simulink model "grua_portuaria"  (R2021a)
settings: Solver=VariableStepAuto  StartTime=0.0  StopTime=2  RelTol=1e-3
values from neighbouring files (symbols this model uses):
  b_cx = 1*10^6    (= 1000000)    [parametros.m]
  b_cy = 1*10^7    (= 10000000)    [parametros.m]
  b_eq = (b_td+b_tm*(r_t^2))/r_td    (= 10803.6)    [parametros.m]
  b_eqh = 2*(b_hd+b_hm*(r_h^2))/r_hd    (= 23253.3333333)    [parametros.m]
  b_ha = b_eqh/r_h - n_h*w_posh*(J_eqh + 0.5*m_l_*r_hd)/r_h    [parametros.m]
  b_hb = 1*10^8    (= 100000000)    [parametros.m]
  b_hEb = 2.2*10^9    (= 2200000000)    [parametros.m]
  b_t = 90    [parametros.m]
  b_ta = n_t*w_post*(r_td*J_eqt/r_t) - r_td*b_eqt/r_t    [parametros.m]
  b_tb = 5*10^6    (= 5000000)    [parametros.m]
  b_tw = 3*10^3    (= 3000)    [parametros.m]
  b_wu = 150    [parametros.m]
  g = 9.80665    [parametros.m]
  H_c = 2.5    [parametros.m]
  J_eq = (J_td+J_tm_tb*(r_t^2))/r_td    (= 15000)    [parametros.m]
  J_eqh = 2*(J_hd_hEb+J_hm_hb*(r_h^2))/r_hd    (= 48853.3333333)    [parametros.m]
  K_cy = 1.8*10^9    (= 1800000000)    [parametros.m]
  K_hsa = -n_h*(w_posh^2)*(J_eqh + 0.5*m_l_*r_hd)/r_t    [parametros.m]
  K_hsia = -(w_posh^3)*(J_eqh + 0.5*m_l_*r_hd)/r_t    [parametros.m]
  K_tsa = n_t*(w_post^2)*J_eqt*r_td/r_t    [parametros.m]
  K_tsia = (w_post^3)*J_eqt*r_td/r_t    [parametros.m]
  K_tw = 4.8*10^5    (= 480000)    [parametros.m]
  k_wu = 2.36*10^8    (= 236000000)    [parametros.m]
  M_s = 15000    [parametros.m]
  M_t = 30000    [parametros.m]
  r_h = 22    [parametros.m]
  r_hd = 0.75    [parametros.m]
  r_t = 30    [parametros.m]
  r_td = 0.5    [parametros.m]
  T_hb_MAX = 5*10^5    (= 500000)    [parametros.m]
  T_hEb_MAX = 1.1*10^6    (= 1100000)    [parametros.m]
  T_s2 = 5e-3    (= 0.005)    [parametros.m]
  T_tb_MAX = 5*10^4    (= 50000)    [parametros.m]
  tau_hm = 1e-3    (= 0.001)    [parametros.m]
  tau_tm = 1e-3    (= 0.001)    [parametros.m]
  Y_t0 = 45    [parametros.m]
undefined symbols (not defined in the file or in its folder): T_s
libraries: simulink x9, dspstat3 x1, vrlib x1
(part 1 of 3)
settings Model: Creator=aguss  LastModifiedBy=Usuario

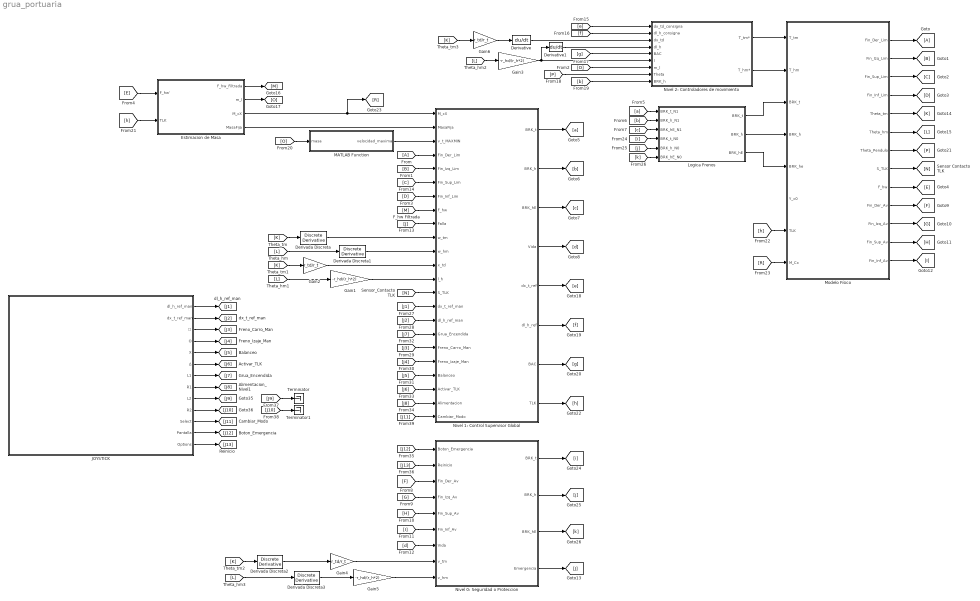
== system grua_portuaria ==
  Derivada Discreta{,1..3} (4 alike) : simulink/Discrete/Discrete Derivative  gainval=1.0  ICPrevScaledInput=0.0  OutMin=[]  OutMax=[]  OutDataType=fixdt(1, 16)  OutScaling=2^-10  DoSatur=off
  Derivative : Derivative
  Derivative1 : Derivative
  Estimacion de Masa : Subsystem
  Gain1 : Gain  Gain=-r_hd/(r_h*2)
  Gain2 : Gain  Gain=r_td/r_t
  Gain3 : Gain  Gain=-r_hd/(r_h*2)
  Gain4 : Gain  Gain=r_td/r_t
  Gain5 : Gain  Gain=-r_hd/(r_h*2)
  Gain6 : Gain  Gain=r_td/r_t
  JOYSTICK : Subsystem
  Logica Frenos : Subsystem
  MATLAB Function : MATLAB Function  TreatAsAtomicUnit=on
  Modelo Físico : Subsystem
  Nivel 0: Seguridad o Proteccion : Subsystem
  Nivel 1: Control Supervisor Global : Subsystem
  Nivel 2: Controladores de movimiento : Subsystem
  Terminator : Terminator
  Terminator1 : Terminator
  wires:
  Nivel 2: Controladores de movimiento/2(T_hm*) -> Modelo Físico/2(T_hm)
  Nivel 2: Controladores de movimiento/1(T_tm*) -> Modelo Físico/1(T_tm)
  Modelo Físico/1(Fin_Der_Lim) -> [A]
  Modelo Físico/2(Fin_Izq_Lim) -> [B]
  Modelo Físico/4(Fin_Inf_Lim) -> [D]
  Modelo Físico/3(Fin_Sup_Lim) -> [C]
  [A] -> Nivel 1: Control Supervisor Global/4(Fin_Der_Lim)
  [B] -> Nivel 1: Control Supervisor Global/5(Fin_Izq_Lim)
  [C] -> Nivel 1: Control Supervisor Global/6(Fin_Sup_Lim)
  [D] -> Nivel 1: Control Supervisor Global/7(Fin_Inf_Lim)
  Modelo Físico/9(F_hw) -> [E]
  Nivel 1: Control Supervisor Global/1(BRK_t) -> [a]
  Nivel 1: Control Supervisor Global/2(BRK_h) -> [b]
  Nivel 1: Control Supervisor Global/3(BRK_hE) -> [c]
  Nivel 1: Control Supervisor Global/4(Vida) -> [d]
  Modelo Físico/10(Fin_Der_Av) -> [F]
  Modelo Físico/11(Fin_Izq_Av) -> [G]
  Modelo Físico/12(Fin_Sup_Av) -> [H]
  Modelo Físico/13(Fin_Inf_Av) -> [I]
  [H] -> Nivel 0: Seguridad o Proteccion/5(Fin_Sup_Av)
  [F] -> Nivel 0: Seguridad o Proteccion/3(Fin_Der_Av)
  [G] -> Nivel 0: Seguridad o Proteccion/4(Fin_Izq_Av)
  [I] -> Nivel 0: Seguridad o Proteccion/6(Fin_Inf_Av)
  [d] -> Nivel 0: Seguridad o Proteccion/7(Vida)
  [E] -> Estimacion de Masa/1(F_hw')
  [M] -> Nivel 1: Control Supervisor Global/8(F_hw)
  Nivel 0: Seguridad o Proteccion/4(Emergencia) -> [J]
  [J] -> Nivel 1: Control Supervisor Global/9(Falla)
  Modelo Físico/5(Theta_tm) -> [K]
  [K] -> Derivada Discreta/1
  Derivada Discreta/1 -> Nivel 1: Control Supervisor Global/10(w_tm)
  Modelo Físico/6(Theta_hm) -> [L]
  [L] -> Derivada Discreta1/1
  Derivada Discreta1/1 -> Nivel 1: Control Supervisor Global/11(w_hm)
  [K] -> Gain2/1
  Gain2/1 -> Nivel 1: Control Supervisor Global/12(x_td)
  [L] -> Gain1/1
  Gain1/1 -> Nivel 1: Control Supervisor Global/13(l_h)
  Estimacion de Masa/4(MasaFija) -> Nivel 1: Control Supervisor Global/2(MasaFija)
  Estimacion de Masa/3(M_cX) -> [R], Nivel 1: Control Supervisor Global/1(M_cX)
  Estimacion de Masa/1(F_hw_Filtrada) -> [M]
  Modelo Físico/8(S_TLK) -> [N]
  [N] -> Nivel 1: Control Supervisor Global/14(S_TLK)
  Estimacion de Masa/2(m_l) -> [O]
  [O] -> Nivel 2: Controladores de movimiento/7(m_l)
  Nivel 1: Control Supervisor Global/5(dx_t_ref) -> [e]
  Nivel 1: Control Supervisor Global/6(dl_h_ref) -> [f]
  Nivel 1: Control Supervisor Global/7(BAC) -> [g]
  [g] -> Nivel 2: Controladores de movimiento/5(BAC)
  [L] -> Gain3/1
  Gain3/1 -> Nivel 2: Controladores de movimiento/6(l), Derivative1/1
  Modelo Físico/7(Theta_Pendulo) -> [P]
  [P] -> Nivel 2: Controladores de movimiento/8(Theta)
  [b] -> Nivel 2: Controladores de movimiento/9(BRK_h)
  MATLAB Function/1(velocidad_maxima) -> Nivel 1: Control Supervisor Global/3(v_t_MAXMIN)
  [O] -> MATLAB Function/1(masa)
  Nivel 1: Control Supervisor Global/8(TLK) -> [h]
  [h] -> Estimacion de Masa/2(TLK)
  [h] -> Modelo Físico/7(TLK)
  [R] -> Modelo Físico/8(M_Cx)
  [a] -> Logica Frenos/1(BRK_t_N1)
  [b] -> Logica Frenos/2(BRK_h_N1)
  [c] -> Logica Frenos/3(BRK_hE_N1)
  Nivel 0: Seguridad o Proteccion/3(BRK_hE) -> [k]
  Nivel 0: Seguridad o Proteccion/2(BRK_h) -> [j]
  Nivel 0: Seguridad o Proteccion/1(BRK_t) -> [i]
  [i] -> Logica Frenos/4(BRK_t_N0)
  [j] -> Logica Frenos/5(BRK_h_N0)
  [k] -> Logica Frenos/6(BRK_hE_N0)
  Logica Frenos/2(BRK_h) -> Modelo Físico/4(BRK_h)
  Logica Frenos/3(BRK_hE) -> Modelo Físico/5(BRK_he)
  Logica Frenos/1(BRK_t) -> Modelo Físico/3(BRK_t)
  [L] -> Derivada Discreta3/1
  Derivada Discreta2/1 -> Gain4/1
  [K] -> Derivada Discreta2/1
  Derivada Discreta3/1 -> Gain5/1
  Gain5/1 -> Nivel 0: Seguridad o Proteccion/9(v_hm)
  Gain4/1 -> Nivel 0: Seguridad o Proteccion/8(v_tm)
  [f] -> Nivel 2: Controladores de movimiento/2(dl_h_consigna)
  [e] -> Nivel 2: Controladores de movimiento/1(dx_td_consigna)
  [K] -> Gain6/1
  Gain6/1 -> Derivative/1
  Derivative/1 -> Nivel 2: Controladores de movimiento/3(dx_td)
  Derivative1/1 -> Nivel 2: Controladores de movimiento/4(dl_h)
  JOYSTICK/1(dl_h_ref_man) -> [J1]
  [J1] -> Nivel 1: Control Supervisor Global/15(dx_t_ref_man)
  [J2] -> Nivel 1: Control Supervisor Global/16(dl_h_ref_man)
  [J3] -> Nivel 1: Control Supervisor Global/18(Freno_Carro_Man)
  [J4] -> Nivel 1: Control Supervisor Global/19(Freno_Izaje_Man)
  JOYSTICK/2(dx_t_ref_man) -> [J2]
  JOYSTICK/3(☐) -> [J3]
  JOYSTICK/4(O) -> [J4]
  [J5] -> Nivel 1: Control Supervisor Global/20(Balanceo)
  [J6] -> Nivel 1: Control Supervisor Global/21(Activar_TLK)
  [J7] -> Nivel 1: Control Supervisor Global/17(Grua_Encendida)
  [J8] -> Nivel 1: Control Supervisor Global/22(Alimentacion)
  [J12] -> Nivel 0: Seguridad o Proteccion/1(Boton_Emergencia)
  [J13] -> Nivel 0: Seguridad o Proteccion/2(Reinicio)
  JOYSTICK/5(X) -> [J5]
  JOYSTICK/6(Δ) -> [J6]
  JOYSTICK/7(L1) -> [J7]
  JOYSTICK/8(R1) -> [J8]
  JOYSTICK/9(L2) -> [J9]
  JOYSTICK/10(R2) -> [J10]
  JOYSTICK/11(Select) -> [J11]
  [J9] -> Terminator/1
  [J10] -> Terminator1/1
  [J11] -> Nivel 1: Control Supervisor Global/23(Cambiar_Modo)
  JOYSTICK/12(Pantalla) -> [J12]
  JOYSTICK/13(Options) -> [J13]

== system grua_portuaria/Estimacion de Masa ==
  F_hw' : Inport
  TLK : Inport  Port=2
  MATLAB Function : MATLAB Function  TreatAsAtomicUnit=on
  Moving Average : dspstat3/Moving Average  Method=Sliding window  ForgettingFactorPort=off  SpecifyWindowLength=on  WindowLength=4  ForgettingFactor=0.9  SimulateUsing=Code generation
  F_hw_Filtrada : Outport
  m_l : Outport  Port=2
  M_cX : Outport  Port=3
  MasaFija : Outport  Port=4
  wires:
  Moving Average/1 -> F_hw_Filtrada/1, MATLAB Function/1(tension)
  F_hw'/1 -> Moving Average/1
  MATLAB Function/3(MasaFija) -> MasaFija/1
  TLK/1 -> MATLAB Function/2(TLK)
  MATLAB Function/2(M_cX) -> M_cX/1
  MATLAB Function/1(m_l) -> m_l/1

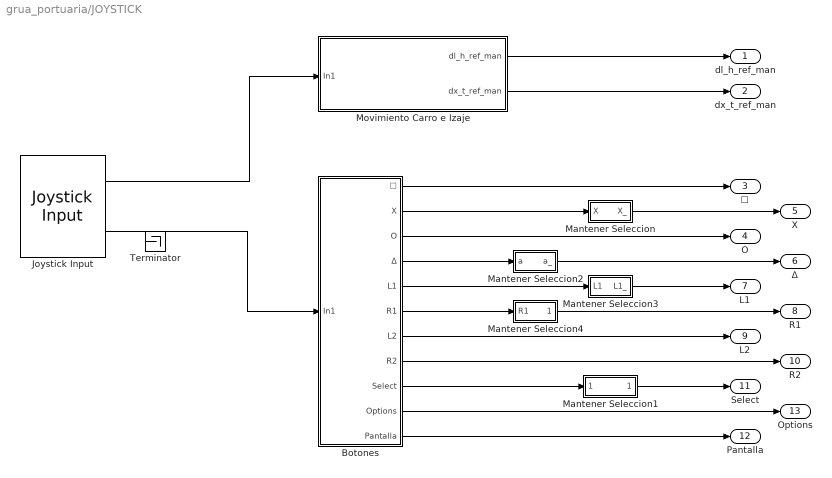
== system grua_portuaria/JOYSTICK ==
  Botones : Subsystem
  Joystick Input : vrlib/Joystick Input  joyid=1  adjustports=on  forcefeed=off
  Mantener Seleccion : Stateflow chart  TreatAsAtomicUnit=on
  Mantener Seleccion1 : Stateflow chart  TreatAsAtomicUnit=on
  Mantener Seleccion2 : Stateflow chart  TreatAsAtomicUnit=on
  Mantener Seleccion3 : Stateflow chart  TreatAsAtomicUnit=on
  Mantener Seleccion4 : Stateflow chart  TreatAsAtomicUnit=on
  Movimiento Carro e Izaje : Subsystem
  Terminator : Terminator
  dl_h_ref_man : Outport
  dx_t_ref_man : Outport  Port=2
  ☐ : Outport  Port=3
  O : Outport  Port=4
  X : Outport  Port=5
  Δ : Outport  Port=6
  L1 : Outport  Port=7
  R1 : Outport  Port=8
  L2 : Outport  Port=9
  R2 : Outport  Port=10
  Select : Outport  Port=11
  Pantalla : Outport  Port=12
  Options : Outport  Port=13
  wires:
  Joystick Input/1 -> Movimiento Carro e Izaje/1(In1)
  Movimiento Carro e Izaje/1(dl_h_ref_man) -> dl_h_ref_man/1
  Movimiento Carro e Izaje/2(dx_t_ref_man) -> dx_t_ref_man/1
  Joystick Input/2 -> Botones/1(In1)
  Botones/1(☐) -> ☐/1
  Botones/2(X) -> Mantener Seleccion/1(X)
  Botones/3(O) -> O/1
  Botones/4(Δ) -> Mantener Seleccion2/1(a)
  Botones/5(L1) -> Mantener Seleccion3/1(L1)
  Botones/6(R1) -> Mantener Seleccion4/1(R1)
  Botones/7(L2) -> L2/1
  Botones/8(R2) -> R2/1
  Botones/9(Select) -> Mantener Seleccion1/1(Select)
  Botones/10(Options) -> Options/1
  Botones/11(Pantalla) -> Pantalla/1
  ? -> Terminator/1
  Mantener Seleccion/1(X_) -> X/1
  Mantener Seleccion2/1(a_) -> Δ/1
  Mantener Seleccion3/1(L1_) -> L1/1
  Mantener Seleccion4/1(R1_) -> R1/1
  Mantener Seleccion1/1(Select_) -> Select/1

== system grua_portuaria/Logica Frenos ==
  BRK_t_N1 : Inport
  BRK_h_N1 : Inport  Port=2
  BRK_hE_N1 : Inport  Port=3
  BRK_t_N0 : Inport  Port=4
  BRK_h_N0 : Inport  Port=5
  BRK_hE_N0 : Inport  Port=6
  AND : Logic  IconShape=distinctive  AllPortsSameDT=off  OutDataTypeStr=boolean
  AND1 : Logic  IconShape=distinctive  AllPortsSameDT=off  OutDataTypeStr=boolean
  AND2 : Logic  IconShape=distinctive  AllPortsSameDT=off  OutDataTypeStr=boolean
  BRK_t : Outport
  BRK_h : Outport  Port=2
  BRK_hE : Outport  Port=3
  wires:
  AND/1 -> BRK_h/1
  BRK_h_N1/1 -> AND/1
  BRK_h_N0/1 -> AND/2
  AND1/1 -> BRK_t/1
  BRK_t_N1/1 -> AND1/1
  BRK_t_N0/1 -> AND1/2
  AND2/1 -> BRK_hE/1
  BRK_hE_N1/1 -> AND2/1
  BRK_hE_N0/1 -> AND2/2

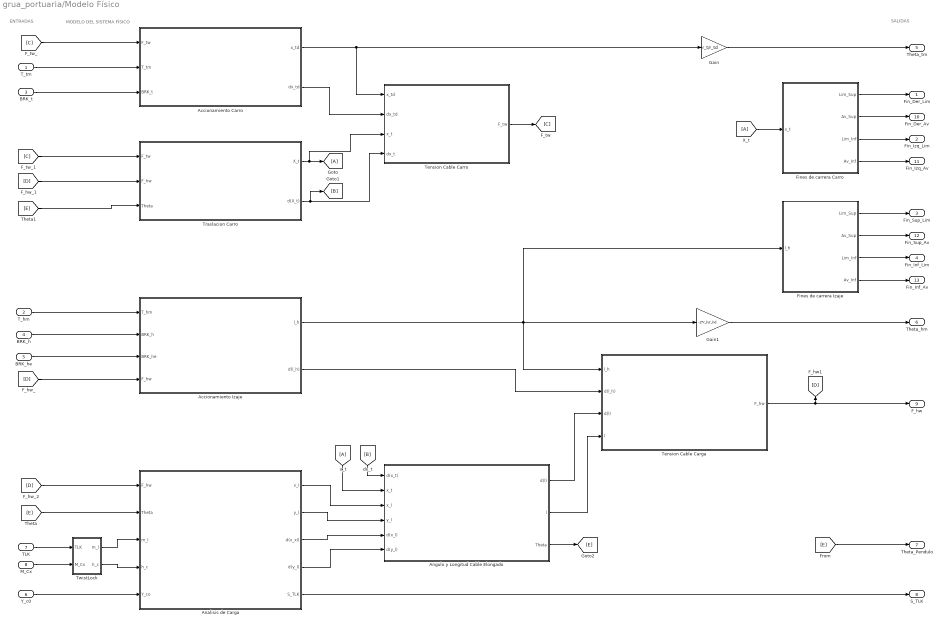
== system grua_portuaria/Modelo Físico ==
  note: SALIDAS
  note: MODELO DEL SISTEMA FÍSICO
  note: ENTRADAS
  T_tm : Inport
  T_hm : Inport  Port=2
  BRK_t : Inport  Port=3
  BRK_h : Inport  Port=4
  BRK_he : Inport  Port=5
  Y_c0 : Inport  Port=6
  TLK : Inport  Port=7
  M_Cx : Inport  Port=8
  Accionamiento Carro : Subsystem
  Accionamiento Izaje : Subsystem
  Analisis de Carga : Subsystem
  Angulo y Longitud Cable Elongado : Subsystem
  Fines de carrera Carro : Subsystem
  Fines de carrera Izaje : Subsystem
  Gain : Gain  Gain=r_t/r_td
  Gain1 : Gain  Gain=-2*r_h/r_hd
  Tension Cable Carga : Subsystem
  Tension Cable Carro : Subsystem
  Traslacion Carro : Subsystem
  TwistLock : Subsystem
  Fin_Der_Lim : Outport
  Fin_Izq_Lim : Outport  Port=2
  Fin_Sup_Lim : Outport  Port=3
  Fin_Inf_Lim : Outport  Port=4
  Theta_tm : Outport  Port=5
  Theta_hm : Outport  Port=6
  Theta_Pendulo : Outport  Port=7
  S_TLK : Outport  Port=8
  F_hw : Outport  Port=9
  Fin_Der_Av : Outport  Port=10
  Fin_Izq_Av : Outport  Port=11
  Fin_Sup_Av : Outport  Port=12
  Fin_Inf_Av : Outport  Port=13
  wires:
  Analisis de Carga/5(S_TLK) -> S_TLK/1
  Fines de carrera Carro/3(Lim_Inf) -> Fin_Izq_Lim/1
  Traslacion Carro/1(X_t) -> Tension Cable Carro/3(x_t), [A]
  Fines de carrera Izaje/2(Av_Sup) -> Fin_Sup_Av/1
  [D] -> Accionamiento Izaje/4(F_hw)
  Angulo y Longitud Cable Elongado/3(Theta) -> [E]
  T_tm/1 -> Accionamiento Carro/2(T_tm)
  Tension Cable Carga/1(F_hw) -> F_hw/1, [D]
  TwistLock/1(m_l) -> Analisis de Carga/3(m_l)
  [E] -> Analisis de Carga/2(Theta)
  Accionamiento Izaje/1(l_h) -> Fines de carrera Izaje/1(l_h), Tension Cable Carga/1(l_h), Gain1/1
  BRK_t/1 -> Accionamiento Carro/3(BRK_t)
  Fines de carrera Carro/1(Lim_Sup) -> Fin_Der_Lim/1
  Accionamiento Carro/1(x_td) -> Gain/1, Tension Cable Carro/1(x_td)
  Fines de carrera Izaje/3(Lim_Inf) -> Fin_Inf_Lim/1
  Analisis de Carga/2(y_l) -> Angulo y Longitud Cable Elongado/4(y_l)
  TwistLock/2(h_c) -> Analisis de Carga/4(h_c)
  BRK_h/1 -> Accionamiento Izaje/2(BRK_h)
  Fines de carrera Carro/2(Av_Sup) -> Fin_Der_Av/1
  [D] -> Analisis de Carga/1(F_hw)
  Accionamiento Carro/2(dx_td) -> Tension Cable Carro/2(dx_td)
  Tension Cable Carro/1(F_tw) -> [C]
  T_hm/1 -> Accionamiento Izaje/1(T_hm)
  [C] -> Accionamiento Carro/1(F_tw)
  [E] -> Theta_Pendulo/1
  Traslacion Carro/2(d(X_t)) -> Tension Cable Carro/4(dx_t), [B]
  [D] -> Traslacion Carro/2(F_hw)
  Y_c0/1 -> Analisis de Carga/5(Y_co)
  Fines de carrera Izaje/4(Av_Inf) -> Fin_Inf_Av/1
  Angulo y Longitud Cable Elongado/1(d(l)) -> Tension Cable Carga/3(d(l))
  M_Cx/1 -> TwistLock/2(M_Cx)
  TLK/1 -> TwistLock/1(TLK)
  [E] -> Traslacion Carro/3(Theta)
  Accionamiento Izaje/2(d(l_h)) -> Tension Cable Carga/2(d(l_h))
  Fines de carrera Izaje/1(Lim_Sup) -> Fin_Sup_Lim/1
  Gain1/1 -> Theta_hm/1
  Fines de carrera Carro/4(Av_Inf) -> Fin_Izq_Av/1
  Angulo y Longitud Cable Elongado/2(l) -> Tension Cable Carga/4(l)
  [B] -> Angulo y Longitud Cable Elongado/1(d(x_t))
  Analisis de Carga/3(d(x_xl)) -> Angulo y Longitud Cable Elongado/5(d(x_l))
  Analisis de Carga/1(x_l) -> Angulo y Longitud Cable Elongado/3(x_l)
  Analisis de Carga/4(d(y_l)) -> Angulo y Longitud Cable Elongado/6(d(y_l))
  Gain/1 -> Theta_tm/1
  [C] -> Traslacion Carro/1(F_tw)
  [A] -> Angulo y Longitud Cable Elongado/2(x_t)
  [A] -> Fines de carrera Carro/1(x_t)
  BRK_he/1 -> Accionamiento Izaje/3(BRK_he)

== system grua_portuaria/Nivel 0: Seguridad o Proteccion ==
  Boton_Emergencia : Inport
  Reinicio : Inport  Port=2
  Fin_Der_Av : Inport  Port=3
  Fin_Izq_Av : Inport  Port=4
  Fin_Sup_Av : Inport  Port=5
  Fin_Inf_Av : Inport  Port=6
  Vida : Inport  Port=7
  v_tm : Inport  Port=8
  v_hm : Inport  Port=9
  Chart : Stateflow chart  TreatAsAtomicUnit=on
  BRK_t : Outport
  BRK_h : Outport  Port=2
  BRK_hE : Outport  Port=3
  Emergencia : Outport  Port=4
  wires:
  Boton_Emergencia/1 -> Chart/1(Boton_Emergencia)
  Chart/1(BRK_t) -> BRK_t/1
  Chart/2(BRK_h) -> BRK_h/1
  Chart/3(BRK_hE) -> BRK_hE/1
  Reinicio/1 -> Chart/2(Reinicio)
  Fin_Der_Av/1 -> Chart/3(Fin_Der_Av)
  Fin_Izq_Av/1 -> Chart/4(Fin_Izq_Av)
  Fin_Sup_Av/1 -> Chart/5(Fin_Sup_Av)
  Fin_Inf_Av/1 -> Chart/6(Fin_Inf_Av)
  Vida/1 -> Chart/7(data)
  Chart/4(Emergencia) -> Emergencia/1
  v_tm/1 -> Chart/8(v_tm)
  v_hm/1 -> Chart/9(v_hm)

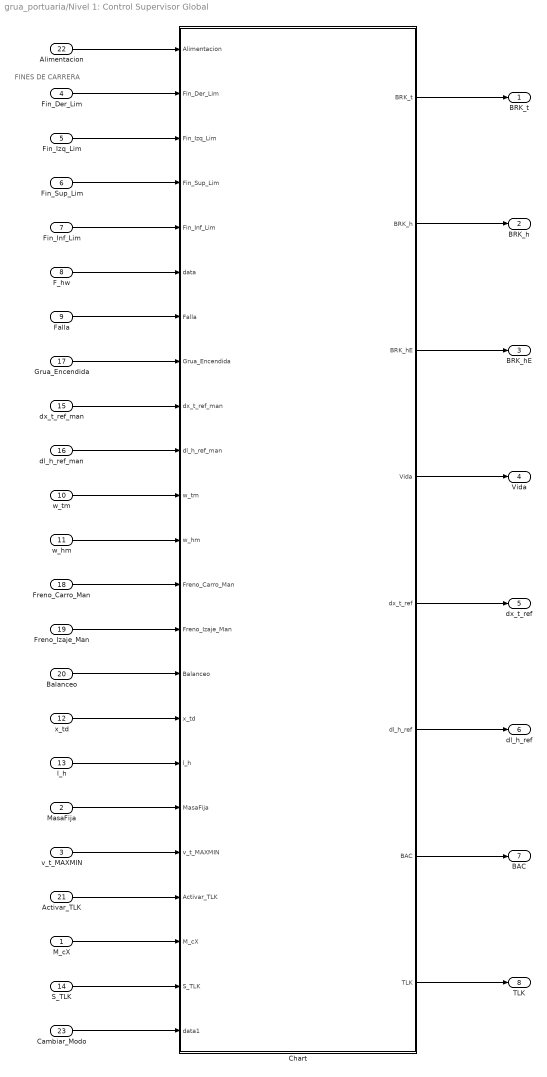
== system grua_portuaria/Nivel 1: Control Supervisor Global ==
  note: FINES DE CARRERA
  M_cX : Inport
  MasaFija : Inport  Port=2
  v_t_MAXMIN : Inport  Port=3
  Fin_Der_Lim : Inport  Port=4
  Fin_Izq_Lim : Inport  Port=5
  Fin_Sup_Lim : Inport  Port=6
  Fin_Inf_Lim : Inport  Port=7
  F_hw : Inport  Port=8
  Falla : Inport  Port=9
  w_tm : Inport  Port=10
  w_hm : Inport  Port=11
  x_td : Inport  Port=12
  l_h : Inport  Port=13
  S_TLK : Inport  Port=14
  dx_t_ref_man : Inport  Port=15
  dl_h_ref_man : Inport  Port=16
  Grua_Encendida : Inport  Port=17
  Freno_Carro_Man : Inport  Port=18
  Freno_Izaje_Man : Inport  Port=19
  Balanceo : Inport  Port=20
  Activar_TLK : Inport  Port=21
  Alimentacion : Inport  Port=22
  Cambiar_Modo : Inport  Port=23
  Chart : Stateflow chart  TreatAsAtomicUnit=on
  BRK_t : Outport
  BRK_h : Outport  Port=2
  BRK_hE : Outport  Port=3
  Vida : Outport  Port=4
  dx_t_ref : Outport  Port=5
  dl_h_ref : Outport  Port=6
  BAC : Outport  Port=7
  TLK : Outport  Port=8
  wires:
  Alimentacion/1 -> Chart/1(Alimentacion)
  Fin_Der_Lim/1 -> Chart/2(Fin_Der_Lim)
  Fin_Izq_Lim/1 -> Chart/3(Fin_Izq_Lim)
  Fin_Sup_Lim/1 -> Chart/4(Fin_Sup_Lim)
  Fin_Inf_Lim/1 -> Chart/5(Fin_Inf_Lim)
  F_hw/1 -> Chart/6(data)
  Chart/1(BRK_t) -> BRK_t/1
  Chart/2(BRK_h) -> BRK_h/1
  Chart/3(BRK_hE) -> BRK_hE/1
  Chart/4(Vida) -> Vida/1
  Falla/1 -> Chart/7(Falla)
  Grua_Encendida/1 -> Chart/8(Grua_Encendida)
  dx_t_ref_man/1 -> Chart/9(dx_t_ref_man)
  dl_h_ref_man/1 -> Chart/10(dl_h_ref_man)
  w_tm/1 -> Chart/11(w_tm)
  w_hm/1 -> Chart/12(w_hm)
  Freno_Carro_Man/1 -> Chart/13(Freno_Carro_Man)
  Freno_Izaje_Man/1 -> Chart/14(Freno_Izaje_Man)
  Balanceo/1 -> Chart/15(Balanceo)
  x_td/1 -> Chart/16(x_td)
  l_h/1 -> Chart/17(l_h)
  MasaFija/1 -> Chart/18(MasaFija)
  v_t_MAXMIN/1 -> Chart/19(v_t_MAXMIN)
  Activar_TLK/1 -> Chart/20(Activar_TLK)
  M_cX/1 -> Chart/21(M_cX)
  S_TLK/1 -> Chart/22(S_TLK)
  Chart/5(dx_t_ref) -> dx_t_ref/1
  Chart/6(dl_h_ref) -> dl_h_ref/1
  Chart/7(BAC) -> BAC/1
  Chart/8(TLK) -> TLK/1
  Cambiar_Modo/1 -> Chart/23(data1)

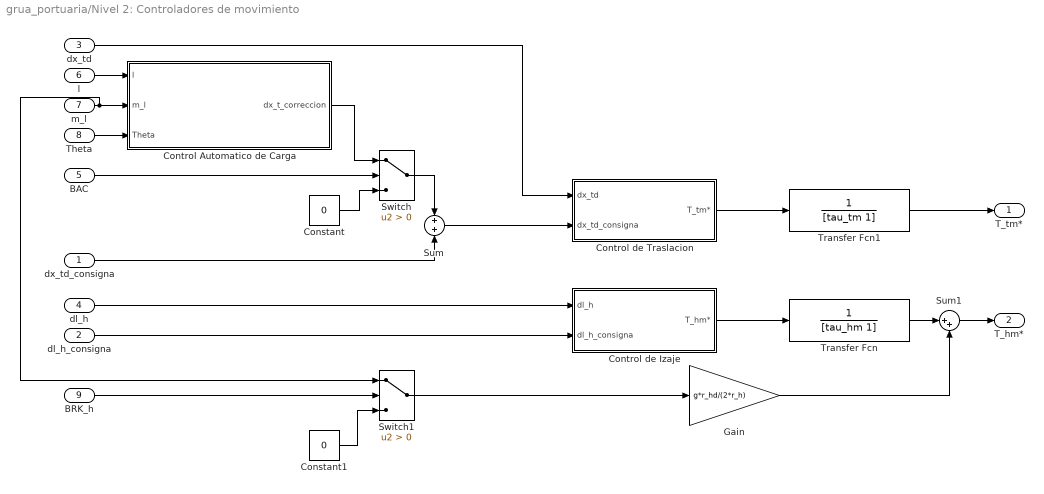
== system grua_portuaria/Nivel 2: Controladores de movimiento ==
  dx_td_consigna : Inport
  dl_h_consigna : Inport  Port=2
  dx_td : Inport  Port=3
  dl_h : Inport  Port=4
  BAC : Inport  Port=5
  l : Inport  Port=6
  m_l : Inport  Port=7
  Theta : Inport  Port=8
  BRK_h : Inport  Port=9
  Constant : Constant  Value=0
  Constant1 : Constant  Value=0
  Control Automatico de Carga : Subsystem
  Control de Izaje : Subsystem
  Control de Traslacion : Subsystem
  Gain : Gain  Gain=g*r_hd/(2*r_h)
  Sum : Sum
  Sum1 : Sum  Inputs=|++
  Switch : Switch  Criteria=u2 > Threshold
  Switch1 : Switch  Criteria=u2 > Threshold
  Transfer Fcn : TransferFcn  Denominator=[tau_hm 1]
  Transfer Fcn1 : TransferFcn  Denominator=[tau_tm 1]
  T_tm* : Outport
  T_hm* : Outport  Port=2
  wires:
  Control de Traslacion/1(T_tm*) -> Transfer Fcn1/1
  Control de Izaje/1(T_hm*) -> Transfer Fcn/1
  dx_td_consigna/1 -> Sum/2
  dx_td/1 -> Control de Traslacion/1(dx_td)
  dl_h/1 -> Control de Izaje/1(dl_h)
  dl_h_consigna/1 -> Control de Izaje/2(dl_h_consigna)
  Sum/1 -> Control de Traslacion/2(dx_td_consigna)
  Control Automatico de Carga/1(dx_t_correccion) -> Switch/1
  Constant/1 -> Switch/3
  Switch/1 -> Sum/1
  BAC/1 -> Switch/2
  Theta/1 -> Control Automatico de Carga/3(Theta)
  m_l/1 -> Control Automatico de Carga/2(m_l), Switch1/1
  l/1 -> Control Automatico de Carga/1(l)
  Transfer Fcn1/1 -> T_tm*/1
  Transfer Fcn/1 -> Sum1/1
  BRK_h/1 -> Switch1/2
  Switch1/1 -> Gain/1
  Constant1/1 -> Switch1/3
  Sum1/1 -> T_hm*/1
  Gain/1 -> Sum1/2

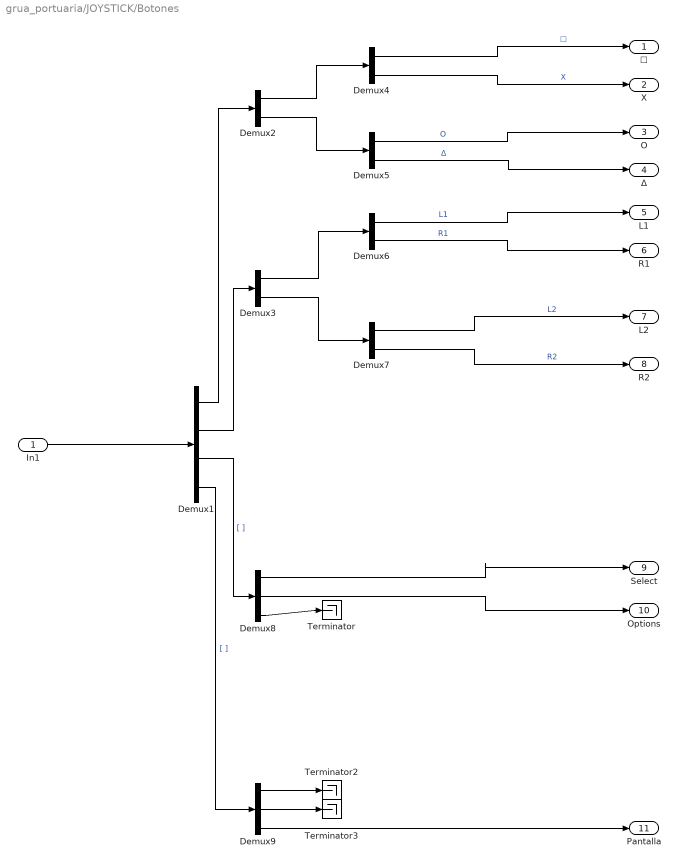
== system grua_portuaria/JOYSTICK/Botones ==
  In1 : Inport
  Demux1 : Demux
  Demux{2..7} (6 alike) : Demux  Outputs=2
  Demux8 : Demux  Outputs=3
  Demux9 : Demux  Outputs=3
  Terminator : Terminator
  Terminator2 : Terminator
  Terminator3 : Terminator
  ☐ : Outport
  X : Outport  Port=2
  O : Outport  Port=3
  Δ : Outport  Port=4
  L1 : Outport  Port=5
  R1 : Outport  Port=6
  L2 : Outport  Port=7
  R2 : Outport  Port=8
  Select : Outport  Port=9
  Options : Outport  Port=10
  Pantalla : Outport  Port=11
  wires:
  Demux6/1 -> L1/1  "L1"
  Demux7/2 -> R2/1  "R2"
  Demux1/2 -> Demux3/1
  Demux1/1 -> Demux2/1
  Demux2/1 -> Demux4/1
  Demux3/2 -> Demux7/1
  Demux2/2 -> Demux5/1
  Demux3/1 -> Demux6/1
  Demux7/1 -> L2/1  "L2"
  Demux4/1 -> ☐/1  "☐"
  Demux5/2 -> Δ/1  "Δ"
  Demux5/1 -> O/1  "O"
  Demux6/2 -> R1/1  "R1"
  Demux4/2 -> X/1  "X"
  Demux1/3 -> Demux8/1  "[ ]"
  In1/1 -> Demux1/1
  Demux8/1 -> Select/1
  Demux8/2 -> Options/1
  Demux8/3 -> Terminator/1
  Demux9/3 -> Pantalla/1
  Demux1/4 -> Demux9/1  "[ ]"
  Demux9/1 -> Terminator2/1
  Demux9/2 -> Terminator3/1

== system grua_portuaria/JOYSTICK/Movimiento Carro e Izaje ==
  In1 : Inport
  Demux : Demux  Outputs=5
  Demux8 : Demux  Outputs=2
  Sensibilidad1 : Subsystem
  Terminator{,2..4} (4 alike) : Terminator
  dl_h_ref_man : Outport
  dx_t_ref_man : Outport  Port=2
  wires:
  Demux8/2 -> Sensibilidad1/1(Analogo_IZQ_Vertical)  "AI_V"
  Demux/3 -> Terminator2/1  "L2"
  Demux/4 -> Terminator3/1  "R2"
  Demux/2 -> Sensibilidad1/2(Analogo_DER_Horizontal)  "AD_H"
  Sensibilidad1/1(dl_h_ref_manual) -> dl_h_ref_man/1
  Sensibilidad1/2(dx_t_ref_man) -> dx_t_ref_man/1
  Demux/5 -> Terminator4/1  "AD_V"
  Demux8/1 -> Terminator/1  "AI_H"
  Demux/1 -> Demux8/1
  In1/1 -> Demux/1

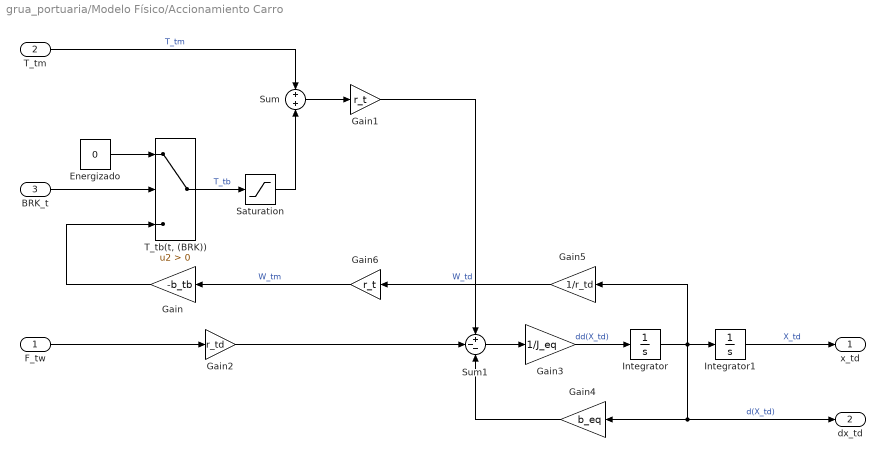
== system grua_portuaria/Modelo Físico/Accionamiento Carro ==
  F_tw : Inport
  T_tm : Inport  Port=2
  BRK_t : Inport  Port=3
  Energizado : Constant  Value=0
  Gain : Gain  Gain=-b_tb
  Gain1 : Gain  Gain=r_t
  Gain2 : Gain  Gain=r_td
  Gain3 : Gain  Gain=1/J_eq
  Gain4 : Gain  Gain=b_eq
  Gain5 : Gain  Gain=1/r_td
  Gain6 : Gain  Gain=r_t
  Integrator : Integrator
  Integrator1 : Integrator
  Saturation : Saturate  UpperLimit=T_tb_MAX  LowerLimit=-T_tb_MAX
  Sum : Sum
  Sum1 : Sum  Inputs=+--
  "T_tb(t, (BRK))" : Switch  Criteria=u2 > Threshold
  x_td : Outport
  dx_td : Outport  Port=2
  wires:
  Energizado/1 -> "T_tb(t, (BRK))"/1
  BRK_t/1 -> "T_tb(t, (BRK))"/2
  Gain/1 -> "T_tb(t, (BRK))"/3
  "T_tb(t, (BRK))"/1 -> Saturation/1  "T_tb"
  T_tm/1 -> Sum/1  "T_tm"
  Sum/1 -> Gain1/1
  Gain1/1 -> Sum1/1
  F_tw/1 -> Gain2/1
  Gain2/1 -> Sum1/2
  Sum1/1 -> Gain3/1
  Gain3/1 -> Integrator/1  "dd(X_td)"
  Integrator/1 -> Gain5/1, dx_td/1, Gain4/1, Integrator1/1  "d(X_td)"
  Integrator1/1 -> x_td/1  "X_td"
  Gain4/1 -> Sum1/3
  Gain5/1 -> Gain6/1  "W_td"
  Gain6/1 -> Gain/1  "W_tm"
  Saturation/1 -> Sum/2

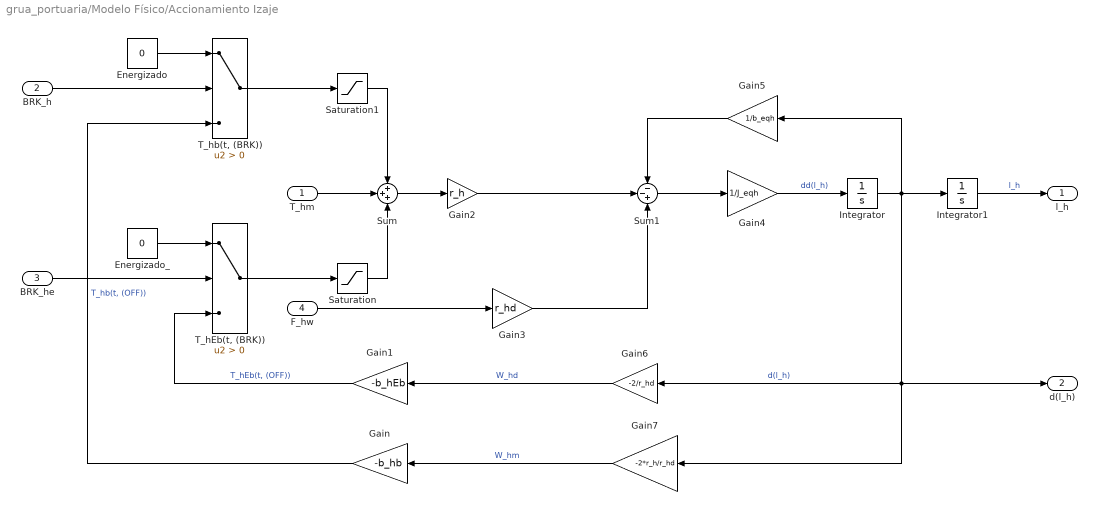
== system grua_portuaria/Modelo Físico/Accionamiento Izaje ==
  T_hm : Inport
  BRK_h : Inport  Port=2
  BRK_he : Inport  Port=3
  F_hw : Inport  Port=4
  Energizado : Constant  Value=0
  Energizado_ : Constant  Value=0
  Gain : Gain  Gain=-b_hb
  Gain1 : Gain  Gain=-b_hEb
  Gain2 : Gain  Gain=r_h
  Gain3 : Gain  Gain=r_hd
  Gain4 : Gain  Gain=1/J_eqh
  Gain5 : Gain  Gain=1/b_eqh
  Gain6 : Gain  Gain=-2/r_hd
  Gain7 : Gain  Gain=-2*r_h/r_hd
  Integrator : Integrator
  Integrator1 : Integrator
  Saturation : Saturate  UpperLimit=T_hEb_MAX  LowerLimit=-T_hEb_MAX
  Saturation1 : Saturate  UpperLimit=T_hb_MAX  LowerLimit=-T_hb_MAX
  Sum : Sum  Inputs=+++
  Sum1 : Sum  Inputs=--+
  "T_hEb(t, (BRK))" : Switch  Criteria=u2 > Threshold
  "T_hb(t, (BRK))" : Switch  Criteria=u2 > Threshold
  l_h : Outport
  d(l_h) : Outport  Port=2
  wires:
  Energizado/1 -> "T_hb(t, (BRK))"/1
  Energizado_/1 -> "T_hEb(t, (BRK))"/1
  BRK_h/1 -> "T_hb(t, (BRK))"/2
  BRK_he/1 -> "T_hEb(t, (BRK))"/2
  Gain/1 -> "T_hb(t, (BRK))"/3  "T_hb(t, (OFF))"
  Gain1/1 -> "T_hEb(t, (BRK))"/3  "T_hEb(t, (OFF))"
  T_hm/1 -> Sum/2
  "T_hb(t, (BRK))"/1 -> Saturation1/1
  "T_hEb(t, (BRK))"/1 -> Saturation/1
  Sum/1 -> Gain2/1
  Gain2/1 -> Sum1/2
  F_hw/1 -> Gain3/1
  Gain3/1 -> Sum1/3
  Sum1/1 -> Gain4/1
  Gain4/1 -> Integrator/1  "dd(l_h)"
  Integrator/1 -> d(l_h)/1, Gain7/1, Gain6/1, Integrator1/1, Gain5/1  "d(l_h)"
  Gain5/1 -> Sum1/1
  Gain6/1 -> Gain1/1  "W_hd"
  Gain7/1 -> Gain/1  "W_hm"
  Integrator1/1 -> l_h/1  "l_h"
  Saturation/1 -> Sum/3
  Saturation1/1 -> Sum/1

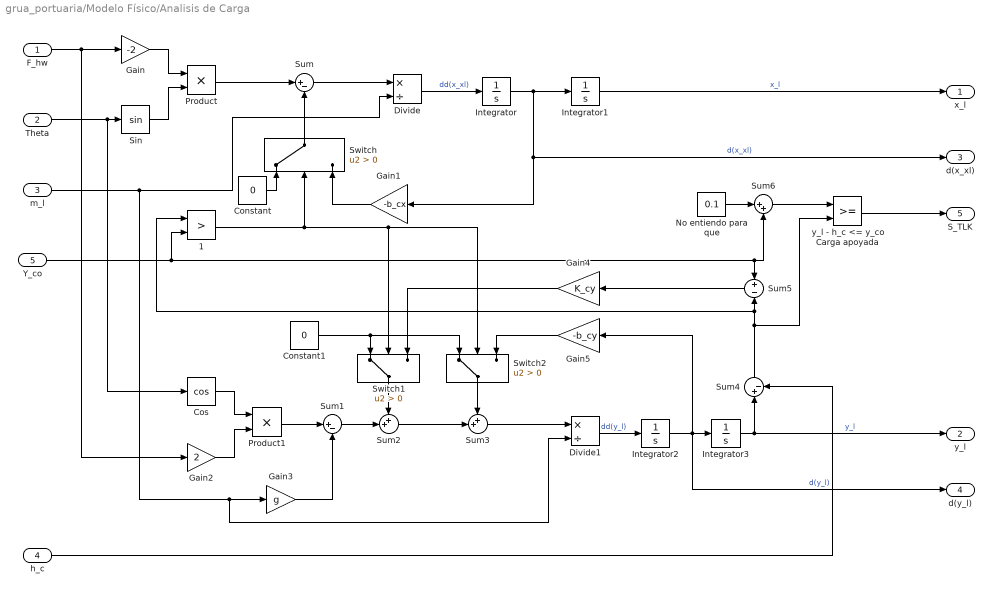
== system grua_portuaria/Modelo Físico/Analisis de Carga ==
  F_hw : Inport
  Theta : Inport  Port=2
  m_l : Inport  Port=3
  h_c : Inport  Port=4
  Y_co : Inport  Port=5
  1 : RelationalOperator  Operator=>  OutDataTypeStr=boolean  RndMeth=Simplest
  Constant : Constant  Value=0
  Constant1 : Constant  Value=0
  Cos : Trigonometry  Operator=cos
  Divide : Product  Inputs=*/
  Divide1 : Product  Inputs=*/
  Gain : Gain  Gain=-2
  Gain1 : Gain  Gain=-b_cx
  Gain2 : Gain  Gain=2
  Gain3 : Gain  Gain=g
  Gain4 : Gain  Gain=K_cy
  Gain5 : Gain  Gain=-b_cy
  Integrator{,1..3} (4 alike) : Integrator
  No entiendo para que : Constant  Value=0.1
  Product : Product
  Product1 : Product
  Sin : Trigonometry
  Sum : Sum  Inputs=|+-
  Sum1 : Sum  Inputs=|+-
  Sum2 : Sum  Inputs=++|
  Sum3 : Sum  Inputs=++|
  Sum4 : Sum  Inputs=|+-
  Sum5 : Sum  Inputs=+-
  Sum6 : Sum  Inputs=|++
  Switch : Switch  Criteria=u2 > Threshold
  Switch1 : Switch  Criteria=u2 > Threshold
  Switch2 : Switch  Criteria=u2 > Threshold
  y_l - h_c <= y_co Carga apoyada : RelationalOperator  OutDataTypeStr=boolean  RndMeth=Simplest
  x_l : Outport
  y_l : Outport  Port=2
  d(x_xl) : Outport  Port=3
  d(y_l) : Outport  Port=4
  S_TLK : Outport  Port=5
  wires:
  F_hw/1 -> Gain2/1, Gain/1
  Theta/1 -> Cos/1, Sin/1
  Gain/1 -> Product/1
  Sin/1 -> Product/2
  Product/1 -> Sum/1
  Constant/1 -> Switch/1
  Gain1/1 -> Switch/3
  Switch/1 -> Sum/2
  Sum/1 -> Divide/1
  m_l/1 -> Divide/2, Divide1/2, Gain3/1
  Divide/1 -> Integrator/1  "dd(x_xl)"
  Integrator/1 -> Integrator1/1, d(x_xl)/1, Gain1/1  "d(x_xl)"
  Integrator1/1 -> x_l/1  "x_l"
  Cos/1 -> Product1/1
  Gain2/1 -> Product1/2
  Gain3/1 -> Sum1/2
  Product1/1 -> Sum1/1
  Constant1/1 -> Switch2/1, Switch1/1
  1/1 -> Switch2/2, Switch1/2, Switch/2
  Gain5/1 -> Switch2/3
  Gain4/1 -> Switch1/3
  Sum3/1 -> Divide1/1
  Switch2/1 -> Sum3/1
  Sum2/1 -> Sum3/2
  Sum1/1 -> Sum2/2
  Switch1/1 -> Sum2/1
  Integrator2/1 -> Gain5/1, d(y_l)/1, Integrator3/1  "d(y_l)"
  Divide1/1 -> Integrator2/1  "dd(y_l)"
  Integrator3/1 -> Sum4/1, y_l/1  "y_l"
  h_c/1 -> Sum4/2
  Sum4/1 -> y_l - h_c <= y_co Carga apoyada/2, 1/1, Sum5/2
  Sum5/1 -> Gain4/1
  Y_co/1 -> 1/2, Sum5/1, Sum6/2
  No entiendo para que/1 -> Sum6/1
  Sum6/1 -> y_l - h_c <= y_co Carga apoyada/1
  y_l - h_c <= y_co Carga apoyada/1 -> S_TLK/1

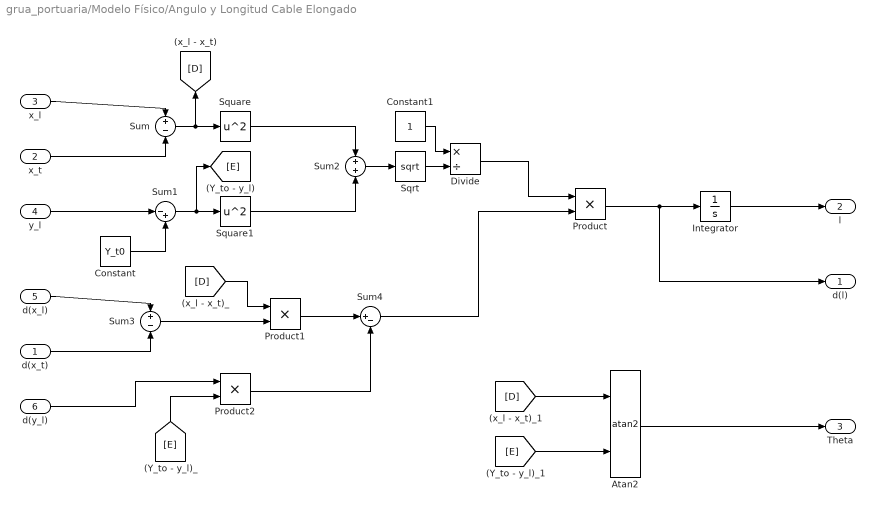
== system grua_portuaria/Modelo Físico/Angulo y Longitud Cable Elongado ==
  d(x_t) : Inport
  x_t : Inport  Port=2
  x_l : Inport  Port=3
  y_l : Inport  Port=4
  d(x_l) : Inport  Port=5
  d(y_l) : Inport  Port=6
  Atan2 : Trigonometry  Operator=atan2
  Constant : Constant  Value=Y_t0
  Constant1 : Constant
  Divide : Product  Inputs=*/
  Integrator : Integrator
  Product : Product
  Product1 : Product
  Product2 : Product
  Sqrt : Sqrt  SaturateOnIntegerOverflow=on
  Square : Math  Operator=square  SaturateOnIntegerOverflow=on
  Square1 : Math  Operator=square  SaturateOnIntegerOverflow=on
  Sum : Sum  Inputs=+-
  Sum1 : Sum  Inputs=|-+
  Sum2 : Sum
  Sum3 : Sum  Inputs=+-
  Sum4 : Sum  Inputs=|+-
  d(l) : Outport
  l : Outport  Port=2
  Theta : Outport  Port=3
  wires:
  x_l/1 -> Sum/1
  x_t/1 -> Sum/2
  Sum/1 -> Square/1, [D]
  y_l/1 -> Sum1/1
  Constant/1 -> Sum1/2
  Sum1/1 -> [E], Square1/1
  Square/1 -> Sum2/1
  Square1/1 -> Sum2/2
  Sum2/1 -> Sqrt/1
  Constant1/1 -> Divide/1
  Divide/1 -> Product/1
  Sqrt/1 -> Divide/2
  d(x_l)/1 -> Sum3/1
  d(x_t)/1 -> Sum3/2
  Sum3/1 -> Product1/2
  [D] -> Product1/1
  Product1/1 -> Sum4/1
  d(y_l)/1 -> Product2/1
  [E] -> Product2/2
  Product2/1 -> Sum4/2
  Sum4/1 -> Product/2
  Product/1 -> d(l)/1, Integrator/1
  Integrator/1 -> l/1
  [D] -> Atan2/1
  [E] -> Atan2/2
  Atan2/1 -> Theta/1

== system grua_portuaria/Modelo Físico/Fines de carrera Carro ==
  x_t : Inport
  Aviso_Inferior : RelationalOperator  Operator=<=  OutDataTypeStr=boolean  RndMeth=Simplest
  Aviso_Superior : RelationalOperator  OutDataTypeStr=boolean  RndMeth=Simplest
  Constant : Constant  Value=50
  Constant1 : Constant  Value=-30
  Constant2 : Constant  Value=51
  Constant3 : Constant  Value=-31
  Limite_Inferior : RelationalOperator  Operator=<=  OutDataTypeStr=boolean  RndMeth=Simplest
  Limite_Superior : RelationalOperator  OutDataTypeStr=boolean  RndMeth=Simplest
  Lim_Sup : Outport
  Av_Sup : Outport  Port=2
  Lim_Inf : Outport  Port=3
  Av_Inf : Outport  Port=4
  wires:
  Constant/1 -> Limite_Superior/2
  Constant1/1 -> Limite_Inferior/2
  Constant2/1 -> Aviso_Superior/2
  Constant3/1 -> Aviso_Inferior/2
  x_t/1 -> Limite_Superior/1, Aviso_Superior/1, Limite_Inferior/1, Aviso_Inferior/1
  Aviso_Superior/1 -> Av_Sup/1
  Limite_Inferior/1 -> Lim_Inf/1
  Aviso_Inferior/1 -> Av_Inf/1
  Limite_Superior/1 -> Lim_Sup/1

== system grua_portuaria/Modelo Físico/Fines de carrera Izaje ==
  l_h : Inport
  Aviso_Inferior : RelationalOperator  Operator=<=  OutDataTypeStr=boolean  RndMeth=Simplest
  Aviso_Superior : RelationalOperator  OutDataTypeStr=boolean  RndMeth=Simplest
  Constant : Constant  Value=40
  Constant1 : Constant  Value=-20
  Constant2 : Constant  Value=41
  Constant3 : Constant  Value=-21
  Constant4 : Constant  Value=Y_t0
  Limite_Inferior : RelationalOperator  Operator=<=  OutDataTypeStr=boolean  RndMeth=Simplest
  Limite_Superior : RelationalOperator  OutDataTypeStr=boolean  RndMeth=Simplest
  x_h = Y_t0 - l_h : Sum  Inputs=|-+
  Lim_Sup : Outport
  Av_Sup : Outport  Port=2
  Lim_Inf : Outport  Port=3
  Av_Inf : Outport  Port=4
  wires:
  Limite_Inferior/1 -> Lim_Inf/1
  Constant/1 -> Limite_Superior/2
  Constant1/1 -> Limite_Inferior/2
  x_h = Y_t0 - l_h/1 -> Limite_Superior/1, Aviso_Superior/1, Limite_Inferior/1, Aviso_Inferior/1
  Limite_Superior/1 -> Lim_Sup/1
  Constant3/1 -> Aviso_Inferior/2
  Aviso_Inferior/1 -> Av_Inf/1
  Aviso_Superior/1 -> Av_Sup/1
  Constant2/1 -> Aviso_Superior/2
  l_h/1 -> x_h = Y_t0 - l_h/1
  Constant4/1 -> x_h = Y_t0 - l_h/2

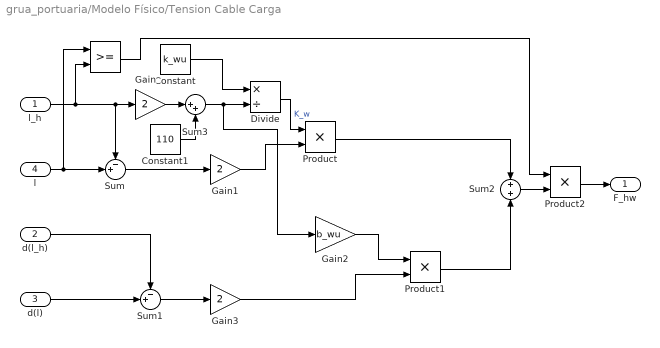
== system grua_portuaria/Modelo Físico/Tension Cable Carga ==
  l_h : Inport
  d(l_h) : Inport  Port=2
  d(l) : Inport  Port=3
  l : Inport  Port=4
  " " : RelationalOperator  OutDataTypeStr=boolean  RndMeth=Simplest
  Constant : Constant  Value=k_wu
  Constant1 : Constant  Value=110
  Divide : Product  Inputs=*/
  Gain : Gain  Gain=2
  Gain1 : Gain  Gain=2
  Gain2 : Gain  Gain=b_wu
  Gain3 : Gain  Gain=2
  Product : Product
  Product1 : Product
  Product2 : Product
  Sum : Sum  Inputs=-+|
  Sum1 : Sum  Inputs=-+|
  Sum2 : Sum
  Sum3 : Sum  Inputs=|++
  F_hw : Outport
  wires:
  l_h/1 -> Gain/1, Sum/1, " "/2
  Sum/1 -> Gain1/1
  Gain1/1 -> Product/2
  d(l)/1 -> Sum1/2
  d(l_h)/1 -> Sum1/1
  Sum1/1 -> Gain3/1
  Gain2/1 -> Product1/1
  Gain3/1 -> Product1/2
  Product/1 -> Sum2/1
  Product1/1 -> Sum2/2
  Constant/1 -> Divide/1
  Gain/1 -> Sum3/1
  Sum3/1 -> Gain2/1, Divide/2
  Constant1/1 -> Sum3/2
  Divide/1 -> Product/1  "K_w"
  l/1 -> " "/1, Sum/2
  Sum2/1 -> Product2/2
  Product2/1 -> F_hw/1
  " "/1 -> Product2/1

== system grua_portuaria/Modelo Físico/Tension Cable Carro ==
  x_td : Inport
  dx_td : Inport  Port=2
  x_t : Inport  Port=3
  dx_t : Inport  Port=4
  Gain : Gain  Gain=K_tw
  Gain1 : Gain  Gain=b_tw
  Sum : Sum  Inputs=+-
  Sum1 : Sum  Inputs=+-
  Sum2 : Sum
  F_tw : Outport
  wires:
  x_td/1 -> Sum/1
  x_t/1 -> Sum/2
  Sum/1 -> Gain/1
  Sum1/1 -> Gain1/1
  dx_td/1 -> Sum1/1
  dx_t/1 -> Sum1/2
  Gain/1 -> Sum2/1
  Gain1/1 -> Sum2/2
  Sum2/1 -> F_tw/1

== system grua_portuaria/Modelo Físico/Traslacion Carro ==
  F_tw : Inport
  F_hw : Inport  Port=2
  Theta : Inport  Port=3
  Gain : Gain  Gain=2
  Gain1 : Gain  Gain=1/M_t
  Gain2 : Gain  Gain=b_t
  Integrator : Integrator
  Integrator1 : Integrator
  Product : Product
  Sin : Trigonometry
  Sum : Sum  Inputs=++-
  X_t : Outport
  d(X_t) : Outport  Port=2
  wires:
  Theta/1 -> Sin/1
  Sin/1 -> Product/2
  F_hw/1 -> Product/1
  Product/1 -> Gain/1
  Gain/1 -> Sum/2
  F_tw/1 -> Sum/1
  Sum/1 -> Gain1/1
  Gain1/1 -> Integrator/1  "dd(X_t)"
  Integrator/1 -> d(X_t)/1, Gain2/1, Integrator1/1  "d(X_t)"
  Gain2/1 -> Sum/3
  Integrator1/1 -> X_t/1

== system grua_portuaria/Modelo Físico/TwistLock ==
  TLK : Inport
  M_Cx : Inport  Port=2
  Chart : Stateflow chart  TreatAsAtomicUnit=on
  Chart1 : Stateflow chart  TreatAsAtomicUnit=on
  Display{,1..3} (4 alike) : Display
  m_l : Outport
  h_c : Outport  Port=2
  wires:
  Chart/1(m_l) -> Display/1, m_l/1
  Chart/2(h_c) -> h_c/1, Display1/1
  M_Cx/1 -> Chart1/2(M_Cx), Chart/2(M_Cx)
  Chart1/1(m_l) -> Display2/1
  Chart1/2(h_c) -> Display3/1
  TLK/1 -> Chart1/1(TLK), Chart/1(TLK)

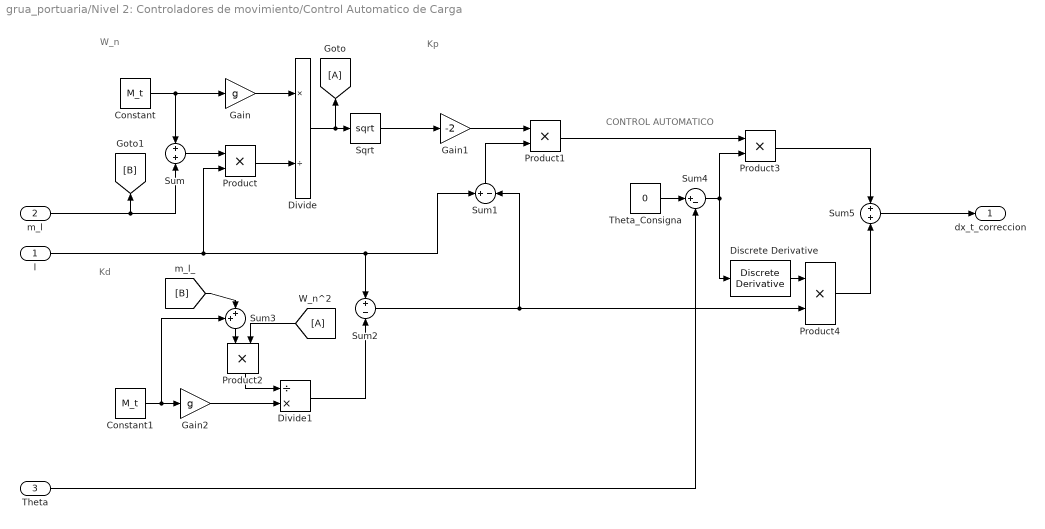
== system grua_portuaria/Nivel 2: Controladores de movimiento/Control Automatico de Carga ==
  note: CONTROL AUTOMATICO
  note: Kd
  note: Kp
  note: W_n
  l : Inport
  m_l : Inport  Port=2
  Theta : Inport  Port=3
  Constant : Constant  Value=M_t
  Constant1 : Constant  Value=M_t
  Discrete Derivative : simulink/Discrete/Discrete Derivative  gainval=1.0  ICPrevScaledInput=0.0  OutMin=[]  OutMax=[]  OutDataType=fixdt(1, 16)  OutScaling=2^-10  DoSatur=off
  Divide : Product  Inputs=*/
  Divide1 : Product  Inputs=/*
  Gain : Gain  Gain=g
  Gain1 : Gain  Gain=-2
  Gain2 : Gain  Gain=g
  Product{,1..4} (5 alike) : Product
  Sqrt : Sqrt  SaturateOnIntegerOverflow=on
  Sum : Sum
  Sum1 : Sum  Inputs=+-
  Sum2 : Sum  Inputs=+-
  Sum3 : Sum  Inputs=++|
  Sum4 : Sum  Inputs=|+-
  Sum5 : Sum
  Theta_Consigna : Constant  Value=0
  dx_t_correccion : Outport
  wires:
  Constant/1 -> Sum/1, Gain/1
  Gain/1 -> Divide/1
  m_l/1 -> [B], Sum/2
  Sum/1 -> Product/1
  l/1 -> Sum1/1, Sum2/1, Product/2
  Product/1 -> Divide/2
  Divide/1 -> [A], Sqrt/1
  Sqrt/1 -> Gain1/1
  Gain1/1 -> Product1/1
  Sum1/1 -> Product1/2
  Constant1/1 -> Sum3/1, Gain2/1
  Gain2/1 -> Divide1/2
  Sum3/1 -> Product2/1
  Product2/1 -> Divide1/1
  [A] -> Product2/2
  [B] -> Sum3/2
  Divide1/1 -> Sum2/2
  Sum2/1 -> Product4/2, Sum1/2
  Theta_Consigna/1 -> Sum4/1
  Theta/1 -> Sum4/2
  Product1/1 -> Product3/1
  Sum4/1 -> Discrete Derivative/1, Product3/2
  Product3/1 -> Sum5/1
  Discrete Derivative/1 -> Product4/1
  Product4/1 -> Sum5/2
  Sum5/1 -> dx_t_correccion/1

== system grua_portuaria/Nivel 2: Controladores de movimiento/Control de Izaje ==
  dl_h : Inport
  dl_h_consigna : Inport  Port=2
  Delay{,1..3} (4 alike) : Delay  DelayLength=1
  Gain : Gain  Gain=b_ha
  Gain1 : Gain  Gain=K_hsa
  Gain2 : Gain  Gain=K_hsia
  Gain3 : Gain  Gain=T_s2/2
  Gain5 : Gain  Gain=T_s2/2
  Sum : Sum  Inputs=-+
  Sum1 : Sum  Inputs=+++
  Sum{2..3,5..6} (4 alike) : Sum  Inputs=|++
  T_hm* : Outport
  wires:
  Delay3/1 -> Sum6/2
  Sum6/1 -> Gain2/1, Delay3/1
  Sum3/1 -> Gain1/1, Delay1/1, Delay2/1, Sum5/1
  Sum5/1 -> Gain5/1
  Gain5/1 -> Sum6/1
  Delay2/1 -> Sum5/2
  Delay1/1 -> Sum3/2
  Gain3/1 -> Sum3/1
  Sum2/1 -> Gain3/1
  Delay/1 -> Sum2/2
  Gain1/1 -> Sum1/2
  Sum1/1 -> T_hm*/1
  dl_h_consigna/1 -> Sum/2
  Sum/1 -> Gain/1, Sum2/1, Delay/1
  dl_h/1 -> Sum/1
  Gain2/1 -> Sum1/1
  Gain/1 -> Sum1/3

== system grua_portuaria/Nivel 2: Controladores de movimiento/Control de Traslacion ==
  dx_td : Inport
  dx_td_consigna : Inport  Port=2
  Delay{,1..3} (4 alike) : Delay  DelayLength=1
  Gain : Gain  Gain=b_ta
  Gain1 : Gain  Gain=K_tsa
  Gain2 : Gain  Gain=K_tsia
  Gain3 : Gain  Gain=T_s/2
  Gain5 : Gain  Gain=T_s/2
  Sum : Sum  Inputs=-+
  Sum1 : Sum  Inputs=+++
  Sum{2..3,5..6} (4 alike) : Sum  Inputs=|++
  T_tm* : Outport
  wires:
  Gain/1 -> Sum1/3
  Gain2/1 -> Sum1/1
  dx_td/1 -> Sum/1
  Sum/1 -> Delay/1, Sum2/1, Gain/1
  dx_td_consigna/1 -> Sum/2
  Sum1/1 -> T_tm*/1
  Gain1/1 -> Sum1/2
  Delay/1 -> Sum2/2
  Sum2/1 -> Gain3/1
  Gain3/1 -> Sum3/1
  Delay1/1 -> Sum3/2
  Delay2/1 -> Sum5/2
  Gain5/1 -> Sum6/1
  Sum5/1 -> Gain5/1
  Sum3/1 -> Sum5/1, Delay2/1, Delay1/1, Gain1/1
  Sum6/1 -> Delay3/1, Gain2/1
  Delay3/1 -> Sum6/2

== system grua_portuaria/JOYSTICK/Movimiento Carro e Izaje/Sensibilidad1 ==
  Analogo_IZQ_Vertical : Inport
  Analogo_DER_Horizontal : Inport  Port=2
  Compare To Constant : simulink/Logic and Bit Operations/Compare To Constant  relop=>=  const=0.15  OutDataTypeStr=boolean
  Compare To Constant1 : simulink/Logic and Bit Operations/Compare To Constant  relop=<=  const=-0.15  OutDataTypeStr=boolean
  Compare To Constant2 : simulink/Logic and Bit Operations/Compare To Constant  relop=>=  const=0.15  OutDataTypeStr=boolean
  Compare To Constant3 : simulink/Logic and Bit Operations/Compare To Constant  relop=<=  const=-0.15  OutDataTypeStr=boolean
  OR : Logic  Operator=OR  IconShape=distinctive  AllPortsSameDT=off  OutDataTypeStr=boolean
  OR1 : Logic  Operator=OR  IconShape=distinctive  AllPortsSameDT=off  OutDataTypeStr=boolean
  Product : Product
  Product1 : Product
  V_max_CARRO : Gain  Gain=4
  V_max_IZAJE : Gain  Gain=3
  dl_h_ref_manual : Outport
  dx_t_ref_man : Outport  Port=2
  wires:
  Analogo_IZQ_Vertical/1 -> V_max_IZAJE/1
  Analogo_DER_Horizontal/1 -> V_max_CARRO/1
  Compare To Constant1/1 -> OR/2
  Compare To Constant2/1 -> OR1/1
  Compare To Constant3/1 -> OR1/2
  OR1/1 -> Product1/1
  Compare To Constant/1 -> OR/1
  OR/1 -> Product/1
  Product/1 -> dl_h_ref_manual/1
  Product1/1 -> dx_t_ref_man/1
  V_max_CARRO/1 -> Product1/2, Compare To Constant2/1, Compare To Constant3/1
  V_max_IZAJE/1 -> Compare To Constant/1, Compare To Constant1/1, Product/2

== stateflow chart grua_portuaria/Modelo Físico/TwistLock/Chart1 ==
  state OFF
    m_l = M_s;
    h_c = 0;
  state ON
    m_l = M_s + M_Cx;
    h_c = H_c;
  (default) -> OFF
  OFF -> ON : [TLK == 1]
  ON -> OFF : [TLK == 0]
  data: TLK input; M_Cx input; m_l output; h_c output; H_c parameter; M_s parameter
